simulink model "TRAS_PID_Cross2"  (Simulink 8.1)
settings: Solver=ode5  SolverMode=SingleTasking  StartTime=0.0  StopTime=90  FixedStep=0.01  RelTol=1e-3  AbsTol=1e-6
undefined symbols (not defined in the file or in its folder): den_FOPID11, den_FOPID22, den_MultiPID_ISE11, den_MultiPID_ISE22, den_MultiPID_ITAE11, den_MultiPID_ITAE22, den_PIDD11, den_PIDD22, den_TFOIDFFID11, den_TFOIDFFID22, den_TID11, den_TID22, num_FOPID11, num_FOPID22, num_MultiPID_ISE11, num_MultiPID_ISE22, num_MultiPID_ITAE11, num_MultiPID_ITAE22, num_PIDD11, num_PIDD22, num_TFOIDFFID11, num_TFOIDFFID22, num_TID11, num_TID22
undefined symbols (not defined in the file): rtdac4pcibaseaddress
libraries: simulink x2
settings Model: Creator=jims  LastModifiedBy=calc2  SimulationMode=external  ExtModeTrigDuration=12000  ExtModeTrigLevel=0.400000
settings DataIOCC: ExternalInput=[]  InitialState=[]  LimitDataPoints=off  MaxDataPoints=5000  SaveOutput=off  SaveTime=off  SignalLoggingName=sigsOut
settings OptimizationCC: BooleanDataType=off  InitFltsAndDblsToZero=on
settings DebuggingCC: SaveWithParameterizedLinksMsg=none  MergeDetectMultiDrivingBlocksExec=error  SolverPrmCheckMsg=none  MultiTaskDSMMsg=warning  MultiTaskCondExecSysMsg=none  IntegerOverflowMsg=none  FcnCallInpInsideContextMsg=EnableAllAsWarning  StrictBusMsg=None
settings HardwareCC: TargetEndianess=LittleEndian  TargetHWDeviceType=MATLAB Host
settings RTWCC: SystemTargetFile=rtwin.tlc  TemplateMakefile=rtwin.tmf  Description=Real-Time Windows Target  ProcessScript=rtwin_make_rtw_hook  IncludeERTFirstTime=on
settings RTWinTargetCC: TargetFcnLib=ansi_tfl_tmw.mat  TargetLibSuffix=_rtwin.lib  TargetPreCompLibLocation=C:\Program Files\MATLAB\R2013a\toolbox\rtw\targets\rtwin\lib\win32  CodeReplacementLibrary=ANSI_C  ModelReferenceCompliant=off  CompOptLevelCompliant=off  RTWinDir=C:/PROGRA~1/MATLAB/R2013a/toolbox/rtw/targets/rtwin  TargetArch=win32

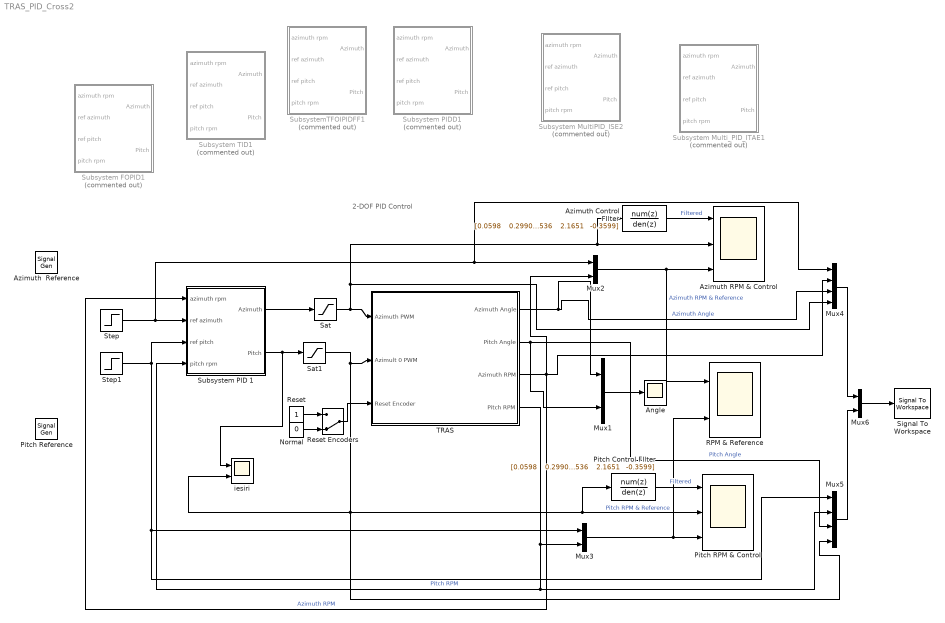
== system TRAS_PID_Cross2 ==
  note: 2-DOF PID Control
  Angle : Scope
      settings: TimeRange=90  YMin=-0.8  YMax=0.5  SaveName=RPM_  MaxDataPoints=12000
  Azimuth RPM & Control : Scope  NumInputPorts=3
      settings: TimeRange=90  YMin=-0.4~-0.5~-2000  YMax=-0.225~0.5~250  SaveName=AngleCtrl_  MaxDataPoints=12000
  Azimuth  Reference : SignalGenerator  WaveForm=square  Amplitude=.8  Frequency=.025
  Azimuth Control FIlter : DiscreteTransferFcn  Numerator="[0.0598    0.2990    0.5980    0.5980    0.2990    0.0598] * 1e-3"  Denominator="[1.0000   -3.9845    6.4349   -5.2536    2.1651   -0.3599]"  SampleTime=0.01
  Mux{1..3,6} (4 alike) : Mux  Inputs=2
  Mux4 : Mux
  Mux5 : Mux
  Normal : Constant  Value=0
  Pitch RPM & Control : Scope  NumInputPorts=3
      settings: TimeRange=90  YMin=2.77556e-17~-0.1~-1300  YMax=0.75~0.9~100  SaveName=AngleCtrl1_  MaxDataPoints=12000
  Pitch Reference : SignalGenerator  Amplitude=.3  Frequency=1/30
  Pitch Control FIlter : DiscreteTransferFcn  Numerator="[0.0598    0.2990    0.5980    0.5980    0.2990    0.0598] * 1e-3"  Denominator="[1.0000   -3.9845    6.4349   -5.2536    2.1651   -0.3599]"  SampleTime=0.01
  RPM & Reference : Scope  NumInputPorts=2
      settings: TimeRange=90  YMin=-1000~-100  YMax=1250~125  SaveName=AngleReference_  MaxDataPoints=12000
  Reset : Constant
  Reset Encoders : ManualSwitch  CurrentSetting=0
  Sat : Saturate
  Sat1 : Saturate  UpperLimit=1  LowerLimit=-.2
  Signal To Workspace : SignalToWorkspace  VariableName=step_pitch
      settings: CopyFcn=dspblkcopystw(gcbh);
  Step : Step  Time=0  After=0  SampleTime=0
  Step1 : Step  Time=0  After=0.5  SampleTime=0
  Subsystem FOPID1 : Subsystem  Commented=on
  Subsystem MultiPID_ISE2 : Subsystem  Commented=on
  Subsystem Multi_PID_ITAE1 : Subsystem  Commented=on
  Subsystem PID 1 : Subsystem
  Subsystem PIDD1 : Subsystem  Commented=on
  Subsystem TID1 : Subsystem  Commented=on
  SubsystemTFOIPIDFF1 : Subsystem  Commented=on
  TRAS : Subsystem  mask{BaseAddress=rtdac4pcibaseaddress, T0=0.01}
      mask prompts: BaseAddress "Base Address:"; T0 "Sampling Period:"
      mask Display: image(imread('TRAS.JPG'))
  iesiri : Scope  NumInputPorts=2
      settings: TimeRange=90  YMin=-0.5~-0.2  YMax=-0.5~-0.2  SaveName=RPM_1  MaxDataPoints=12000
  wires:
  Pitch Control FIlter/1 -> Pitch RPM & Control/1  "Filtered"
  Mux3/1 -> Pitch RPM & Control/3, RPM & Reference/2  "Pitch RPM & Reference"
  TRAS/2(Pitch Angle) -> Mux1/2, Mux5/3  "Pitch Angle"
  Mux1/1 -> Angle/1
  Sat/1 -> Mux4/4, Azimuth RPM & Control/2, Azimuth Control FIlter/1, TRAS/1(Azimuth PWM)
  Step1/1 -> Mux5/1, Mux3/1, Subsystem PID 1/3(ref pitch)
  Azimuth Control FIlter/1 -> Azimuth RPM & Control/1  "Filtered"
  Mux2/1 -> Azimuth RPM & Control/3, RPM & Reference/1  "Azimuth RPM & Reference"
  Reset Encoders/1 -> TRAS/3(Reset Encoder)
  Reset/1 -> Reset Encoders/1
  Normal/1 -> Reset Encoders/2
  TRAS/4(Pitch RPM) -> Mux3/2, Subsystem PID 1/4(pitch rpm), Mux5/2  "Pitch RPM"
  TRAS/3(Azimuth RPM) -> Subsystem PID 1/1(azimuth rpm), Mux2/2, Mux4/2  "Azimuth RPM"
  TRAS/1(Azimuth Angle) -> Mux1/1, Mux4/3  "Azimuth Angle"
  Subsystem PID 1/1(Azimuth) -> Sat/1
  Subsystem PID 1/2(Pitch) -> iesiri/1, Sat1/1
  Sat1/1 -> Mux5/4, iesiri/2, Pitch RPM & Control/2, Pitch Control FIlter/1, TRAS/2(Azimult 0 PWM)
  Mux4/1 -> Mux6/1
  Mux5/1 -> Mux6/2
  Mux6/1 -> Signal To Workspace/1
  Step/1 -> Subsystem PID 1/2(ref azimuth), Mux2/1, Mux4/1

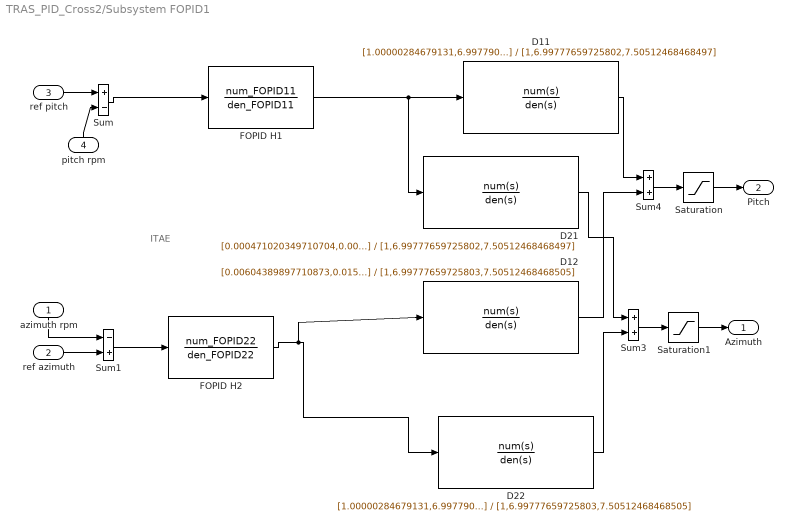
== system TRAS_PID_Cross2/Subsystem FOPID1 ==
  note: ITAE
  azimuth rpm : Inport
  ref azimuth : Inport  Port=2
  ref pitch : Inport  Port=3
  pitch rpm : Inport  Port=4
  D11 : TransferFcn  Numerator=[1.00000284679131,6.99779030125994,7.50513760323875]  Denominator=[1,6.99777659725802,7.50512468468497]
  D12 : TransferFcn  Numerator=[0.00604389897710873,0.0157679645959730,0.0102823375259034]  Denominator=[1,6.99777659725803,7.50512468468505]
  D21 : TransferFcn  Numerator=[0.000471020349710704,0.00433466168519442,0.00942932713768640]  Denominator=[1,6.99777659725802,7.50512468468497]
  D22 : TransferFcn  Numerator=[1.00000284679131,6.99779030126001,7.50513760323899]  Denominator=[1,6.99777659725803,7.50512468468505]
  FOPID H1 : TransferFcn  Numerator=num_FOPID11  Denominator=den_FOPID11
  FOPID H2 : TransferFcn  Numerator=num_FOPID22  Denominator=den_FOPID22
  Saturation : Saturate
  Saturation1 : Saturate  UpperLimit=1  LowerLimit=-0.2
  Sum : Sum  Inputs=+-  SaturateOnIntegerOverflow=on
  Sum1 : Sum  Inputs=-+  SaturateOnIntegerOverflow=on
  Sum3 : Sum  SaturateOnIntegerOverflow=on
  Sum4 : Sum  SaturateOnIntegerOverflow=on
  Azimuth : Outport
  Pitch : Outport  Port=2
  wires:
  D11/1 -> Sum4/1
  D22/1 -> Sum3/2
  FOPID H2/1 -> D22/1, D12/1
  FOPID H1/1 -> D11/1, D21/1
  D12/1 -> Sum4/2
  Saturation1/1 -> Azimuth/1
  Saturation/1 -> Pitch/1
  Sum4/1 -> Saturation/1
  Sum3/1 -> Saturation1/1
  pitch rpm/1 -> Sum/2
  ref pitch/1 -> Sum/1
  ref azimuth/1 -> Sum1/2
  azimuth rpm/1 -> Sum1/1
  Sum/1 -> FOPID H1/1
  Sum1/1 -> FOPID H2/1
  D21/1 -> Sum3/1

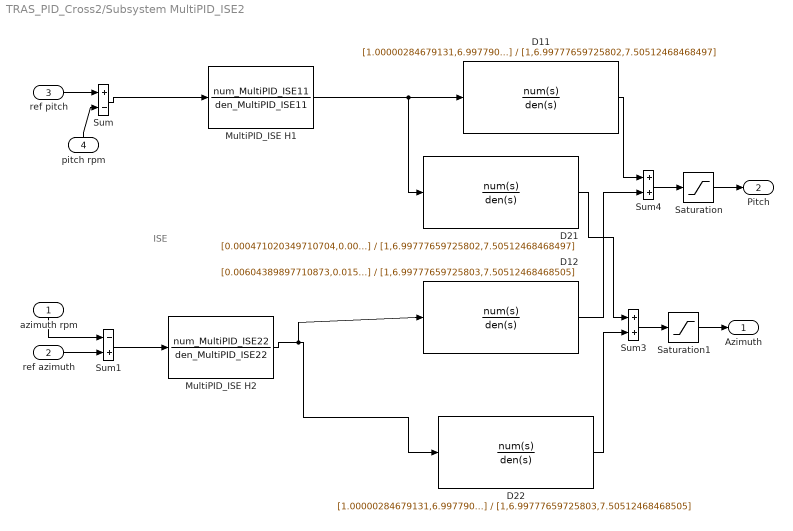
== system TRAS_PID_Cross2/Subsystem MultiPID_ISE2 ==
  note: ISE
  azimuth rpm : Inport
  ref azimuth : Inport  Port=2
  ref pitch : Inport  Port=3
  pitch rpm : Inport  Port=4
  D11 : TransferFcn  Numerator=[1.00000284679131,6.99779030125994,7.50513760323875]  Denominator=[1,6.99777659725802,7.50512468468497]
  D12 : TransferFcn  Numerator=[0.00604389897710873,0.0157679645959730,0.0102823375259034]  Denominator=[1,6.99777659725803,7.50512468468505]
  D21 : TransferFcn  Numerator=[0.000471020349710704,0.00433466168519442,0.00942932713768640]  Denominator=[1,6.99777659725802,7.50512468468497]
  D22 : TransferFcn  Numerator=[1.00000284679131,6.99779030126001,7.50513760323899]  Denominator=[1,6.99777659725803,7.50512468468505]
  MultiPID_ISE H1 : TransferFcn  Numerator=num_MultiPID_ISE11  Denominator=den_MultiPID_ISE11
  MultiPID_ISE H2 : TransferFcn  Numerator=num_MultiPID_ISE22  Denominator=den_MultiPID_ISE22
  Saturation : Saturate
  Saturation1 : Saturate  UpperLimit=1  LowerLimit=-0.2
  Sum : Sum  Inputs=+-  SaturateOnIntegerOverflow=on
  Sum1 : Sum  Inputs=-+  SaturateOnIntegerOverflow=on
  Sum3 : Sum  SaturateOnIntegerOverflow=on
  Sum4 : Sum  SaturateOnIntegerOverflow=on
  Azimuth : Outport
  Pitch : Outport  Port=2
  wires:
  D21/1 -> Sum3/1
  Sum1/1 -> MultiPID_ISE H2/1
  Sum/1 -> MultiPID_ISE H1/1
  azimuth rpm/1 -> Sum1/1
  ref azimuth/1 -> Sum1/2
  ref pitch/1 -> Sum/1
  pitch rpm/1 -> Sum/2
  Sum3/1 -> Saturation1/1
  Sum4/1 -> Saturation/1
  Saturation/1 -> Pitch/1
  Saturation1/1 -> Azimuth/1
  D12/1 -> Sum4/2
  MultiPID_ISE H1/1 -> D21/1, D11/1
  MultiPID_ISE H2/1 -> D12/1, D22/1
  D22/1 -> Sum3/2
  D11/1 -> Sum4/1

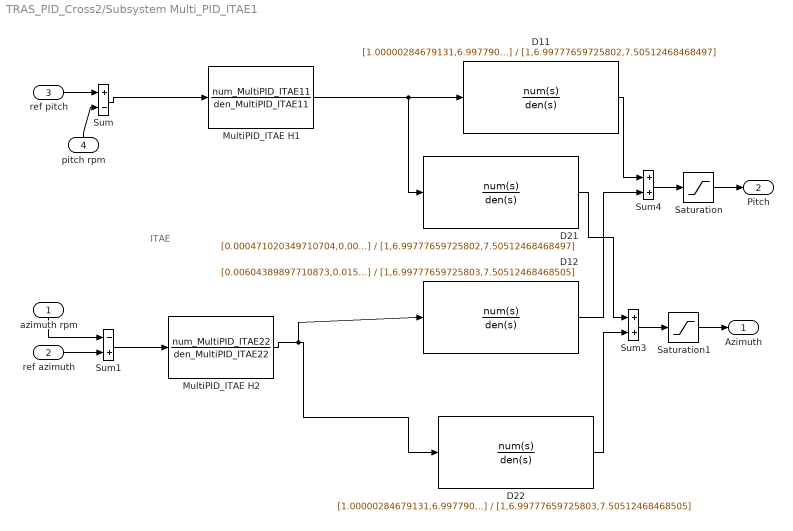
== system TRAS_PID_Cross2/Subsystem Multi_PID_ITAE1 ==
  note: ITAE
  azimuth rpm : Inport
  ref azimuth : Inport  Port=2
  ref pitch : Inport  Port=3
  pitch rpm : Inport  Port=4
  D11 : TransferFcn  Numerator=[1.00000284679131,6.99779030125994,7.50513760323875]  Denominator=[1,6.99777659725802,7.50512468468497]
  D12 : TransferFcn  Numerator=[0.00604389897710873,0.0157679645959730,0.0102823375259034]  Denominator=[1,6.99777659725803,7.50512468468505]
  D21 : TransferFcn  Numerator=[0.000471020349710704,0.00433466168519442,0.00942932713768640]  Denominator=[1,6.99777659725802,7.50512468468497]
  D22 : TransferFcn  Numerator=[1.00000284679131,6.99779030126001,7.50513760323899]  Denominator=[1,6.99777659725803,7.50512468468505]
  MultiPID_ITAE H1 : TransferFcn  Numerator=num_MultiPID_ITAE11  Denominator=den_MultiPID_ITAE11
  MultiPID_ITAE H2 : TransferFcn  Numerator=num_MultiPID_ITAE22  Denominator=den_MultiPID_ITAE22
  Saturation : Saturate
  Saturation1 : Saturate  UpperLimit=1  LowerLimit=-0.2
  Sum : Sum  Inputs=+-  SaturateOnIntegerOverflow=on
  Sum1 : Sum  Inputs=-+  SaturateOnIntegerOverflow=on
  Sum3 : Sum  SaturateOnIntegerOverflow=on
  Sum4 : Sum  SaturateOnIntegerOverflow=on
  Azimuth : Outport
  Pitch : Outport  Port=2
  wires:
  D11/1 -> Sum4/1
  D22/1 -> Sum3/2
  MultiPID_ITAE H2/1 -> D22/1, D12/1
  MultiPID_ITAE H1/1 -> D11/1, D21/1
  D12/1 -> Sum4/2
  Saturation1/1 -> Azimuth/1
  Saturation/1 -> Pitch/1
  Sum4/1 -> Saturation/1
  Sum3/1 -> Saturation1/1
  pitch rpm/1 -> Sum/2
  ref pitch/1 -> Sum/1
  ref azimuth/1 -> Sum1/2
  azimuth rpm/1 -> Sum1/1
  Sum/1 -> MultiPID_ITAE H1/1
  Sum1/1 -> MultiPID_ITAE H2/1
  D21/1 -> Sum3/1

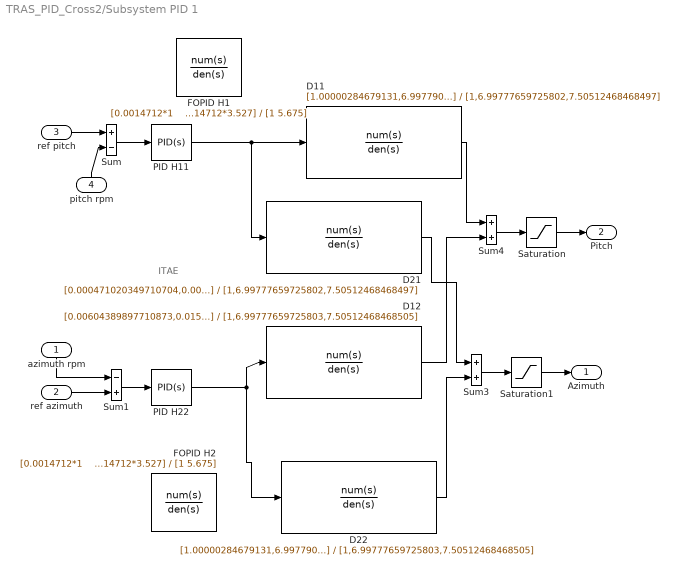
== system TRAS_PID_Cross2/Subsystem PID 1 ==
  note: ITAE
  azimuth rpm : Inport
  ref azimuth : Inport  Port=2
  ref pitch : Inport  Port=3
  pitch rpm : Inport  Port=4
  D11 : TransferFcn  Numerator=[1.00000284679131,6.99779030125994,7.50513760323875]  Denominator=[1,6.99777659725802,7.50512468468497]
  D12 : TransferFcn  Numerator=[0.00604389897710873,0.0157679645959730,0.0102823375259034]  Denominator=[1,6.99777659725803,7.50512468468505]
  D21 : TransferFcn  Numerator=[0.000471020349710704,0.00433466168519442,0.00942932713768640]  Denominator=[1,6.99777659725802,7.50512468468497]
  D22 : TransferFcn  Numerator=[1.00000284679131,6.99779030126001,7.50513760323899]  Denominator=[1,6.99777659725803,7.50512468468505]
  FOPID H1 : TransferFcn  Numerator="[0.0014712*1    0.0014712*3.527]"  Denominator=[1 5.675]
  FOPID H2 : TransferFcn  Numerator="[0.0014712*1    0.0014712*3.527]"  Denominator=[1 5.675]
  PID H11 : simulink/Continuous/PID Controller  Controller=PID  TimeDomain=Continuous-time  SampleTime=1  IntegratorMethod=Forward Euler  FilterMethod=Forward Euler  Form=Parallel  P=0.595  I=0.765  D=0  N=100  InitialConditionSource=internal  InitialConditionForIntegrator=0  InitialConditionForFilter=0  ExternalReset=none  LimitOutput=off  UpperSaturationLimit=inf  LowerSaturationLimit=-inf  LinearizeAsGain=off  AntiWindupMode=none  Kb=1  TrackingMode=off  Kt=1  PParamMin=[]  PParamMax=[]  IParamMin=[]  IParamMax=[]  DParamMin=[]  DParamMax=[]  NParamMin=[]  NParamMax=[]  KbParamMin=[]  KbParamMax=[]  KtParamMin=[]  KtParamMax=[]  POutMin=[]  POutMax=[]  IOutMin=[]  IOutMax=[]  DOutMin=[]  DOutMax=[]  NOutMin=[]  NOutMax=[]  KbOutMin=[]  KbOutMax=[]  KtOutMin=[]  KtOutMax=[]  IntegratorOutMin=[]  IntegratorOutMax=[]  FilterOutMin=[]  FilterOutMax=[]  SumOutMin=[]  SumOutMax=[]  SumI1OutMin=[]  SumI1OutMax=[]  SumI2OutMin=[]  SumI2OutMax=[]  SumI3OutMin=[]  SumI3OutMax=[]  SumDOutMin=[]  SumDOutMax=[]  SaturationOutMin=[]  SaturationOutMax=[]  IntegratorContinuousStateAttributes=''  IntegratorStateMustResolveToSignalObject=off  IntegratorRTWStateStorageClass=Auto  FilterContinuousStateAttributes=''  FilterStateMustResolveToSignalObject=off  FilterRTWStateStorageClass=Auto
  PID H22 : simulink/Continuous/PID Controller  Controller=PID  TimeDomain=Continuous-time  SampleTime=1  IntegratorMethod=Forward Euler  FilterMethod=Forward Euler  Form=Parallel  P=0.067  I=51.1  D=0  N=100  InitialConditionSource=internal  InitialConditionForIntegrator=0  InitialConditionForFilter=0  ExternalReset=none  LimitOutput=off  UpperSaturationLimit=inf  LowerSaturationLimit=-inf  LinearizeAsGain=off  AntiWindupMode=none  Kb=1  TrackingMode=off  Kt=1  PParamMin=[]  PParamMax=[]  IParamMin=[]  IParamMax=[]  DParamMin=[]  DParamMax=[]  NParamMin=[]  NParamMax=[]  KbParamMin=[]  KbParamMax=[]  KtParamMin=[]  KtParamMax=[]  POutMin=[]  POutMax=[]  IOutMin=[]  IOutMax=[]  DOutMin=[]  DOutMax=[]  NOutMin=[]  NOutMax=[]  KbOutMin=[]  KbOutMax=[]  KtOutMin=[]  KtOutMax=[]  IntegratorOutMin=[]  IntegratorOutMax=[]  FilterOutMin=[]  FilterOutMax=[]  SumOutMin=[]  SumOutMax=[]  SumI1OutMin=[]  SumI1OutMax=[]  SumI2OutMin=[]  SumI2OutMax=[]  SumI3OutMin=[]  SumI3OutMax=[]  SumDOutMin=[]  SumDOutMax=[]  SaturationOutMin=[]  SaturationOutMax=[]  IntegratorContinuousStateAttributes=''  IntegratorStateMustResolveToSignalObject=off  IntegratorRTWStateStorageClass=Auto  FilterContinuousStateAttributes=''  FilterStateMustResolveToSignalObject=off  FilterRTWStateStorageClass=Auto
  Saturation : Saturate
  Saturation1 : Saturate  UpperLimit=1  LowerLimit=-0.2
  Sum : Sum  Inputs=+-  SaturateOnIntegerOverflow=on
  Sum1 : Sum  Inputs=-+  SaturateOnIntegerOverflow=on
  Sum3 : Sum  SaturateOnIntegerOverflow=on
  Sum4 : Sum  SaturateOnIntegerOverflow=on
  Azimuth : Outport
  Pitch : Outport  Port=2
  wires:
  D21/1 -> Sum3/1
  Sum1/1 -> PID H22/1
  Sum/1 -> PID H11/1
  azimuth rpm/1 -> Sum1/1
  ref azimuth/1 -> Sum1/2
  ref pitch/1 -> Sum/1
  pitch rpm/1 -> Sum/2
  Sum3/1 -> Saturation1/1
  Sum4/1 -> Saturation/1
  Saturation/1 -> Pitch/1
  Saturation1/1 -> Azimuth/1
  D12/1 -> Sum4/2
  PID H11/1 -> D21/1, D11/1
  PID H22/1 -> D12/1, D22/1
  D22/1 -> Sum3/2
  D11/1 -> Sum4/1

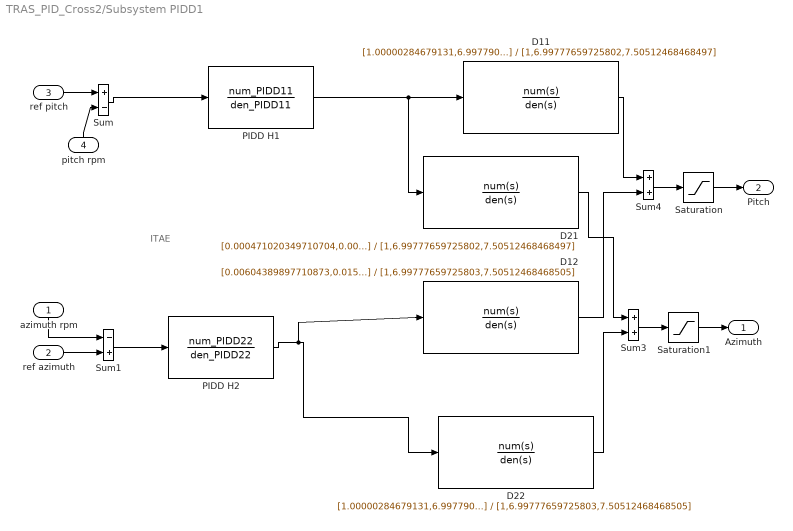
== system TRAS_PID_Cross2/Subsystem PIDD1 ==
  note: ITAE
  azimuth rpm : Inport
  ref azimuth : Inport  Port=2
  ref pitch : Inport  Port=3
  pitch rpm : Inport  Port=4
  D11 : TransferFcn  Numerator=[1.00000284679131,6.99779030125994,7.50513760323875]  Denominator=[1,6.99777659725802,7.50512468468497]
  D12 : TransferFcn  Numerator=[0.00604389897710873,0.0157679645959730,0.0102823375259034]  Denominator=[1,6.99777659725803,7.50512468468505]
  D21 : TransferFcn  Numerator=[0.000471020349710704,0.00433466168519442,0.00942932713768640]  Denominator=[1,6.99777659725802,7.50512468468497]
  D22 : TransferFcn  Numerator=[1.00000284679131,6.99779030126001,7.50513760323899]  Denominator=[1,6.99777659725803,7.50512468468505]
  PIDD H1 : TransferFcn  Numerator=num_PIDD11  Denominator=den_PIDD11
  PIDD H2 : TransferFcn  Numerator=num_PIDD22  Denominator=den_PIDD22
  Saturation : Saturate
  Saturation1 : Saturate  UpperLimit=1  LowerLimit=-0.2
  Sum : Sum  Inputs=+-  SaturateOnIntegerOverflow=on
  Sum1 : Sum  Inputs=-+  SaturateOnIntegerOverflow=on
  Sum3 : Sum  SaturateOnIntegerOverflow=on
  Sum4 : Sum  SaturateOnIntegerOverflow=on
  Azimuth : Outport
  Pitch : Outport  Port=2
  wires:
  D21/1 -> Sum3/1
  Sum1/1 -> PIDD H2/1
  Sum/1 -> PIDD H1/1
  azimuth rpm/1 -> Sum1/1
  ref azimuth/1 -> Sum1/2
  ref pitch/1 -> Sum/1
  pitch rpm/1 -> Sum/2
  Sum3/1 -> Saturation1/1
  Sum4/1 -> Saturation/1
  Saturation/1 -> Pitch/1
  Saturation1/1 -> Azimuth/1
  D12/1 -> Sum4/2
  PIDD H1/1 -> D21/1, D11/1
  PIDD H2/1 -> D12/1, D22/1
  D22/1 -> Sum3/2
  D11/1 -> Sum4/1

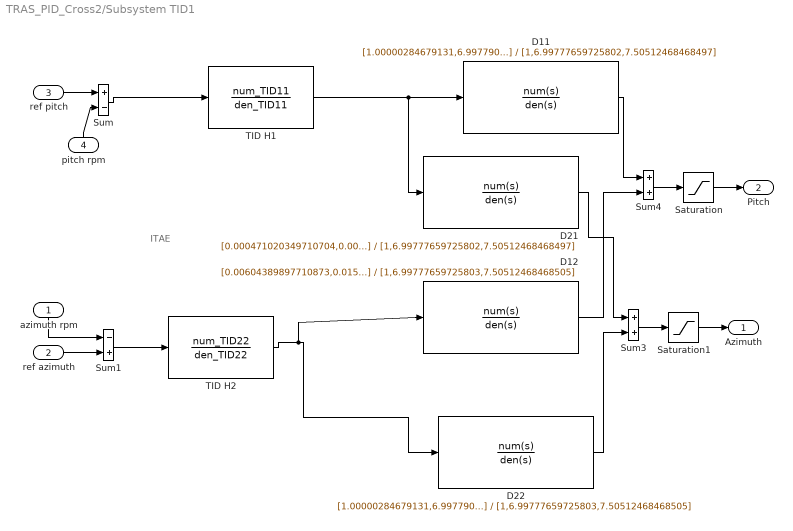
== system TRAS_PID_Cross2/Subsystem TID1 ==
  note: ITAE
  azimuth rpm : Inport
  ref azimuth : Inport  Port=2
  ref pitch : Inport  Port=3
  pitch rpm : Inport  Port=4
  D11 : TransferFcn  Numerator=[1.00000284679131,6.99779030125994,7.50513760323875]  Denominator=[1,6.99777659725802,7.50512468468497]
  D12 : TransferFcn  Numerator=[0.00604389897710873,0.0157679645959730,0.0102823375259034]  Denominator=[1,6.99777659725803,7.50512468468505]
  D21 : TransferFcn  Numerator=[0.000471020349710704,0.00433466168519442,0.00942932713768640]  Denominator=[1,6.99777659725802,7.50512468468497]
  D22 : TransferFcn  Numerator=[1.00000284679131,6.99779030126001,7.50513760323899]  Denominator=[1,6.99777659725803,7.50512468468505]
  Saturation : Saturate
  Saturation1 : Saturate  UpperLimit=1  LowerLimit=-0.2
  Sum : Sum  Inputs=+-  SaturateOnIntegerOverflow=on
  Sum1 : Sum  Inputs=-+  SaturateOnIntegerOverflow=on
  Sum3 : Sum  SaturateOnIntegerOverflow=on
  Sum4 : Sum  SaturateOnIntegerOverflow=on
  TID H1 : TransferFcn  Numerator=num_TID11  Denominator=den_TID11
  TID H2 : TransferFcn  Numerator=num_TID22  Denominator=den_TID22
  Azimuth : Outport
  Pitch : Outport  Port=2
  wires:
  D11/1 -> Sum4/1
  D22/1 -> Sum3/2
  TID H2/1 -> D22/1, D12/1
  TID H1/1 -> D11/1, D21/1
  D12/1 -> Sum4/2
  Saturation1/1 -> Azimuth/1
  Saturation/1 -> Pitch/1
  Sum4/1 -> Saturation/1
  Sum3/1 -> Saturation1/1
  pitch rpm/1 -> Sum/2
  ref pitch/1 -> Sum/1
  ref azimuth/1 -> Sum1/2
  azimuth rpm/1 -> Sum1/1
  Sum/1 -> TID H1/1
  Sum1/1 -> TID H2/1
  D21/1 -> Sum3/1

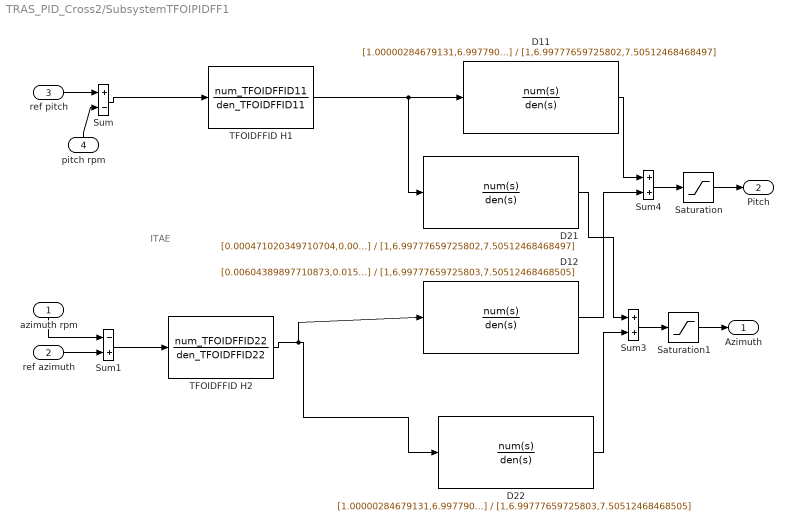
== system TRAS_PID_Cross2/SubsystemTFOIPIDFF1 ==
  note: ITAE
  azimuth rpm : Inport
  ref azimuth : Inport  Port=2
  ref pitch : Inport  Port=3
  pitch rpm : Inport  Port=4
  D11 : TransferFcn  Numerator=[1.00000284679131,6.99779030125994,7.50513760323875]  Denominator=[1,6.99777659725802,7.50512468468497]
  D12 : TransferFcn  Numerator=[0.00604389897710873,0.0157679645959730,0.0102823375259034]  Denominator=[1,6.99777659725803,7.50512468468505]
  D21 : TransferFcn  Numerator=[0.000471020349710704,0.00433466168519442,0.00942932713768640]  Denominator=[1,6.99777659725802,7.50512468468497]
  D22 : TransferFcn  Numerator=[1.00000284679131,6.99779030126001,7.50513760323899]  Denominator=[1,6.99777659725803,7.50512468468505]
  Saturation : Saturate
  Saturation1 : Saturate  UpperLimit=1  LowerLimit=-0.2
  Sum : Sum  Inputs=+-  SaturateOnIntegerOverflow=on
  Sum1 : Sum  Inputs=-+  SaturateOnIntegerOverflow=on
  Sum3 : Sum  SaturateOnIntegerOverflow=on
  Sum4 : Sum  SaturateOnIntegerOverflow=on
  TFOIDFFID H1 : TransferFcn  Numerator=num_TFOIDFFID11  Denominator=den_TFOIDFFID11
  TFOIDFFID H2 : TransferFcn  Numerator=num_TFOIDFFID22  Denominator=den_TFOIDFFID22
  Azimuth : Outport
  Pitch : Outport  Port=2
  wires:
  D11/1 -> Sum4/1
  D22/1 -> Sum3/2
  TFOIDFFID H2/1 -> D22/1, D12/1
  TFOIDFFID H1/1 -> D11/1, D21/1
  D12/1 -> Sum4/2
  Saturation1/1 -> Azimuth/1
  Saturation/1 -> Pitch/1
  Sum4/1 -> Saturation/1
  Sum3/1 -> Saturation1/1
  pitch rpm/1 -> Sum/2
  ref pitch/1 -> Sum/1
  ref azimuth/1 -> Sum1/2
  azimuth rpm/1 -> Sum1/1
  Sum/1 -> TFOIDFFID H1/1
  Sum1/1 -> TFOIDFFID H2/1
  D21/1 -> Sum3/1

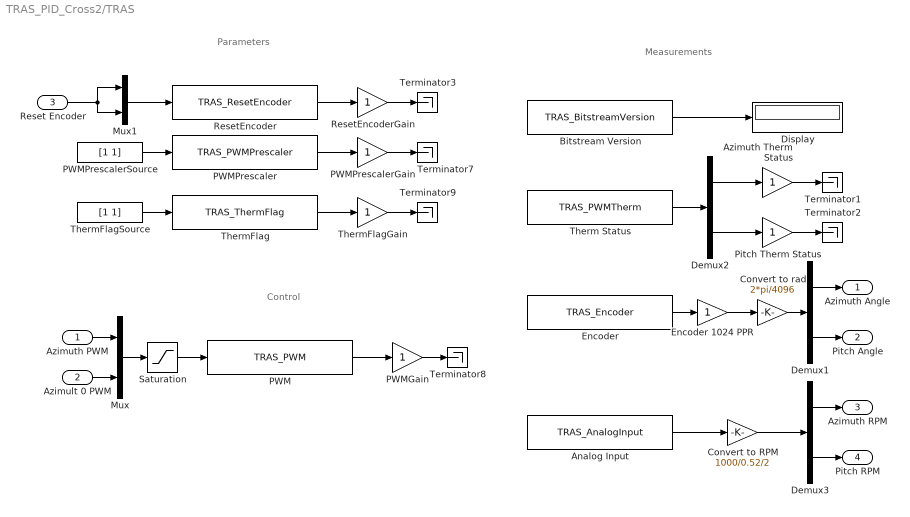
== system TRAS_PID_Cross2/TRAS ==
  note: Parameters
  note: Control
  note: Measurements
  Azimuth PWM : Inport
  Azimult 0 PWM : Inport  Port=2
  Reset Encoder : Inport  Port=3
  Analog Input : S-Function  FunctionName=TRAS_AnalogInput  Parameters=BaseAddress, [1 0], [1 1], T0  EnableBusSupport=off
  Azimuth Therm Status : Gain  SaturateOnIntegerOverflow=on  OutDataTypeStr=Inherit: Same as input  ParamDataTypeStr=Inherit: Same as input
  Bitstream Version : S-Function  FunctionName=TRAS_BitstreamVersion  Parameters=BaseAddress, T0  EnableBusSupport=off
  Convert to RPM : Gain  Gain=1000/0.52/2  SaturateOnIntegerOverflow=on  OutDataTypeStr=Inherit: Same as input  ParamDataTypeStr=Inherit: Same as input
  Convert to rad : Gain  Gain=2*pi/4096  SaturateOnIntegerOverflow=on  OutDataTypeStr=Inherit: Same as input  ParamDataTypeStr=Inherit: Same as input
  Demux1 : Demux  Outputs=2
  Demux2 : Demux  Outputs=2
  Demux3 : Demux  Outputs=2
  Display : Display
  Encoder : S-Function  FunctionName=TRAS_Encoder  Parameters=BaseAddress, T0  EnableBusSupport=off
  Encoder 1024 PPR : Gain  SaturateOnIntegerOverflow=on  OutDataTypeStr=Inherit: Same as input  ParamDataTypeStr=Inherit: Same as input
  Mux : Mux  Inputs=2
  Mux1 : Mux  Inputs=2
  PWM : S-Function  FunctionName=TRAS_PWM  Parameters=BaseAddress, T0  EnableBusSupport=off
  PWMGain : Gain  SaturateOnIntegerOverflow=on  OutDataTypeStr=Inherit: Same as input  ParamDataTypeStr=Inherit: Same as input
  PWMPrescaler : S-Function  FunctionName=TRAS_PWMPrescaler  Parameters=BaseAddress, T0  EnableBusSupport=off
  PWMPrescalerGain : Gain  SaturateOnIntegerOverflow=on  OutDataTypeStr=Inherit: Same as input  ParamDataTypeStr=Inherit: Same as input
  PWMPrescalerSource : Constant  Value=[1 1]
  Pitch Therm Status : Gain  SaturateOnIntegerOverflow=on  OutDataTypeStr=Inherit: Same as input  ParamDataTypeStr=Inherit: Same as input
  ResetEncoder : S-Function  FunctionName=TRAS_ResetEncoder  Parameters=BaseAddress, T0  EnableBusSupport=off
  ResetEncoderGain : Gain  SaturateOnIntegerOverflow=on  OutDataTypeStr=Inherit: Same as input  ParamDataTypeStr=Inherit: Same as input
  Saturation : Saturate  UpperLimit=1  LowerLimit=-1
  Terminator{1..3,7..9} (6 alike) : Terminator
  Therm Status : S-Function  FunctionName=TRAS_PWMTherm  Parameters=BaseAddress, T0  EnableBusSupport=off
  "ThermFlag " : S-Function  FunctionName=TRAS_ThermFlag  Parameters=BaseAddress, T0  EnableBusSupport=off
  ThermFlagGain : Gain  SaturateOnIntegerOverflow=on  OutDataTypeStr=Inherit: Same as input  ParamDataTypeStr=Inherit: Same as input
  ThermFlagSource : Constant  Value=[1 1]
  Azimuth Angle : Outport  InitialOutput=0
  Pitch Angle : Outport  Port=2  InitialOutput=0
  Azimuth RPM : Outport  Port=3  InitialOutput=0
  Pitch RPM : Outport  Port=4  InitialOutput=0
  wires:
  Encoder 1024 PPR/1 -> Convert to rad/1
  Encoder/1 -> Encoder 1024 PPR/1
  Saturation/1 -> PWM/1
  Mux/1 -> Saturation/1
  PWM/1 -> PWMGain/1
  PWMGain/1 -> Terminator8/1
  ResetEncoder/1 -> ResetEncoderGain/1
  PWMPrescaler/1 -> PWMPrescalerGain/1
  Mux1/1 -> ResetEncoder/1
  PWMPrescalerSource/1 -> PWMPrescaler/1
  ResetEncoderGain/1 -> Terminator3/1
  PWMPrescalerGain/1 -> Terminator7/1
  Azimult 0 PWM/1 -> Mux/2
  Azimuth PWM/1 -> Mux/1
  Demux1/2 -> Pitch Angle/1
  Convert to rad/1 -> Demux1/1
  Demux1/1 -> Azimuth Angle/1
  Therm Status/1 -> Demux2/1
  Demux2/2 -> Pitch Therm Status/1
  Demux2/1 -> Azimuth Therm Status/1
  Azimuth Therm Status/1 -> Terminator1/1
  Pitch Therm Status/1 -> Terminator2/1
  Bitstream Version/1 -> Display/1
  Analog Input/1 -> Convert to RPM/1
  Demux3/2 -> Pitch RPM/1
  Demux3/1 -> Azimuth RPM/1
  Reset Encoder/1 -> Mux1/1, Mux1/2
  Convert to RPM/1 -> Demux3/1
  "ThermFlag "/1 -> ThermFlagGain/1
  ThermFlagSource/1 -> "ThermFlag "/1
  ThermFlagGain/1 -> Terminator9/1
